simulink model "envModel_rl"  (R2020b)
settings: Solver=ode23t  StartTime=0.0  StopTime=Tf  RelTol=1e-2
values from neighbouring files (symbols this model uses):
  simlen = 100    [main_rl.m]    (also in main_rl_func_modified.m; new_main_rl.m = 80)
  Tf = 200    [RLenv.m]    (also in RlEnvModel.m; demo_rl.m; main_rl.m = simlen*Ts; main_rl_func_modified.m = simlen*Ts)
  Ts = 0.1    [RLenv.m]    (also in RlEnvModel.m; demo_rl.m; main_rl.m = s.Ts; main_rl_func_modified.m = s.Ts)
  ulim = s.actuatorRange    [main_rl.m]    (also in main_rl_func_modified.m; new_main_rl.m)
  whichAg_sim = whichAg_sim*5    (= 30)    [main_rl.m]    (also in main_rl_func_modified.m; new_main_rl.m)
  ylim = s.sensorRange    [main_rl.m]    (also in main_rl_func_modified.m; new_main_rl.m)
undefined symbols (not defined in the file or in its folder): s
libraries: rllib x3, simulink x2
settings Model: Creator=The MathWorks, Inc.  LastModifiedBy=Asus

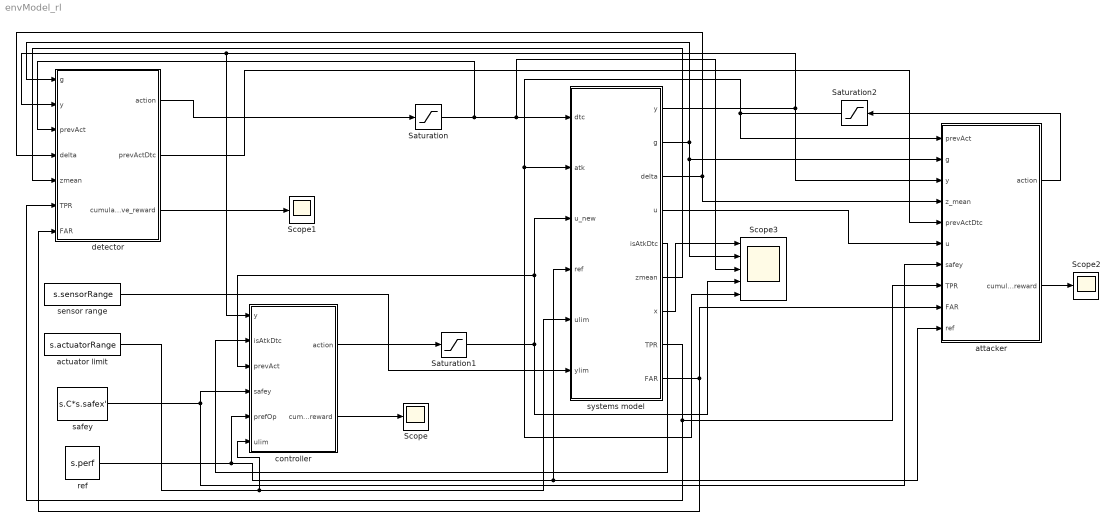
== system envModel_rl ==
  Saturation : Saturate  UpperLimit=[100;simlen]  LowerLimit=[0;1]
  Saturation1 : Saturate  UpperLimit=s.actuatorRange  LowerLimit=-s.actuatorRange
  Saturation2 : Saturate  UpperLimit=[ulim;ylim]  LowerLimit=-[ulim;ylim]
  Scope : Scope
  Scope1 : Scope
  Scope2 : Scope
  Scope3 : Scope  NumInputPorts=5
  actuator limit : Constant  Value=s.actuatorRange
  attacker : Subsystem
  controller : Subsystem
  detector : Subsystem
  ref : Constant  Value=s.perf
  safey : Constant  Value=s.C*s.safex'
  sensor range : Constant  Value=s.sensorRange
  systems model : Subsystem
  wires:
  systems model/1(y) -> controller/1(y), detector/2(y), attacker/3(y)
  ref/1 -> attacker/10(ref), systems model/4(ref), controller/5(prefOp)
  safey/1 -> attacker/7(safey), controller/4(safey)
  systems model/3(delta) -> detector/4(delta), attacker/4(z_mean)
  systems model/2(g) -> detector/1(g), Scope3/2, attacker/2(g)
  sensor range/1 -> systems model/6(ylim)
  actuator limit/1 -> controller/6(ulim), systems model/5(ulim)
  Saturation/1 -> detector/3(prevAct), Scope3/3, systems model/1(dtc)
  Saturation1/1 -> systems model/3(u_new), controller/3(prevAct), Scope3/4
  Saturation2/1 -> attacker/1(prevAct), systems model/2(atk), Scope3/5
  systems model/7(x) -> Scope3/1
  systems model/9(FAR) -> attacker/9(FAR), detector/7(FAR)
  systems model/8(TPR) -> attacker/8(TPR), detector/6(TPR)
  systems model/6(zmean) -> detector/5(zmean)
  detector/1(action) -> Saturation/1
  detector/3(cumulative_reward) -> Scope1/1
  systems model/5(isAtkDtc) -> controller/2(isAtkDtc)
  controller/1(action) -> Saturation1/1
  controller/2(cumulative_reward) -> Scope/1
  detector/2(prevActDtc) -> attacker/5(prevActDtc)
  systems model/4(u) -> attacker/6(u)
  attacker/1(action) -> Saturation2/1
  attacker/2(cumulative_reward) -> Scope2/1

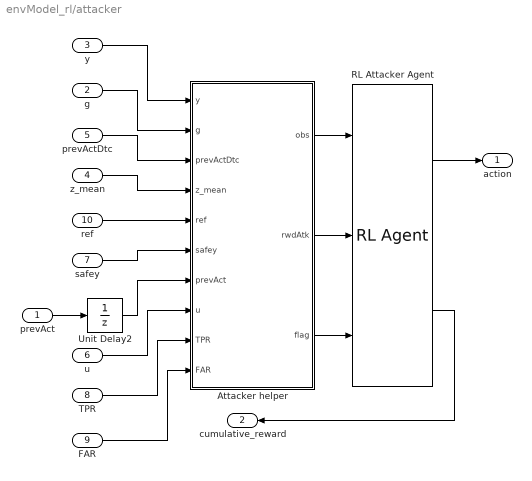
== system envModel_rl/attacker ==
  prevAct : Inport
  g : Inport  Port=2
  y : Inport  Port=3
  z_mean : Inport  Port=4
  prevActDtc : Inport  Port=5
  u : Inport  Port=6
  safey : Inport  Port=7
  TPR : Inport  Port=8
  FAR : Inport  Port=9
  ref : Inport  Port=10
  Attacker helper : Subsystem
  RL Attacker Agent : rllib/RL Agent  Agent=agentAtk  ProvideReward=on  ProvideIsDone=on  ProvideCumRwd=on  TreatAsDirectFeedthrough=on  CollectLoggedSignals=on  CollectModelStates=on
  Unit Delay2 : UnitDelay  SampleTime=-1  HasFrameUpgradeWarning=on
  action : Outport
  cumulative_reward : Outport  Port=2
  wires:
  z_mean/1 -> Attacker helper/4(z_mean)
  prevAct/1 -> Unit Delay2/1
  y/1 -> Attacker helper/1(y)
  ref/1 -> Attacker helper/5(ref)
  Attacker helper/3(flag) -> RL Attacker Agent/3
  Attacker helper/1(obs) -> RL Attacker Agent/1
  Attacker helper/2(rwdAtk) -> RL Attacker Agent/2
  RL Attacker Agent/2 -> cumulative_reward/1
  Unit Delay2/1 -> Attacker helper/7(prevAct)
  RL Attacker Agent/1 -> action/1
  TPR/1 -> Attacker helper/9(TPR)
  FAR/1 -> Attacker helper/10(FAR)
  prevActDtc/1 -> Attacker helper/3(prevActDtc)
  g/1 -> Attacker helper/2(g)
  u/1 -> Attacker helper/8(u)
  safey/1 -> Attacker helper/6(safey)

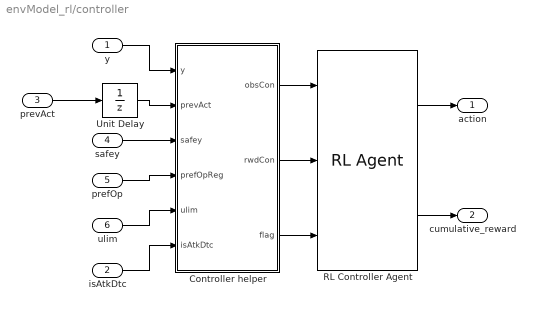
== system envModel_rl/controller ==
  y : Inport
  isAtkDtc : Inport  Port=2
  prevAct : Inport  Port=3
  safey : Inport  Port=4
  prefOp : Inport  Port=5
  ulim : Inport  Port=6
  Controller helper : Subsystem
  RL Controller Agent : rllib/RL Agent  Agent=agentCon  ProvideReward=on  ProvideIsDone=on  ProvideCumRwd=on  TreatAsDirectFeedthrough=on  CollectLoggedSignals=on  CollectModelStates=on
  Unit Delay : UnitDelay  SampleTime=-1  HasFrameUpgradeWarning=on
  action : Outport
  cumulative_reward : Outport  Port=2
  wires:
  Unit Delay/1 -> Controller helper/2(prevAct)
  RL Controller Agent/2 -> cumulative_reward/1
  prefOp/1 -> Controller helper/4(prefOpReg)
  Controller helper/1(obsCon) -> RL Controller Agent/1
  ulim/1 -> Controller helper/5(ulim)
  Controller helper/3(flag) -> RL Controller Agent/3
  safey/1 -> Controller helper/3(safey)
  prevAct/1 -> Unit Delay/1
  Controller helper/2(rwdCon) -> RL Controller Agent/2
  isAtkDtc/1 -> Controller helper/6(isAtkDtc)
  RL Controller Agent/1 -> action/1
  y/1 -> Controller helper/1(y)

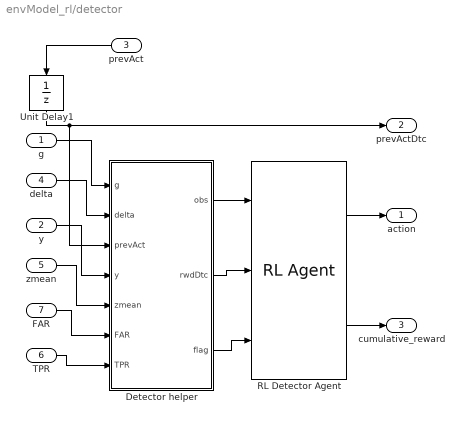
== system envModel_rl/detector ==
  g : Inport
  y : Inport  Port=2
  prevAct : Inport  Port=3
  delta : Inport  Port=4
  zmean : Inport  Port=5
  TPR : Inport  Port=6
  FAR : Inport  Port=7
  Detector helper : Subsystem
  RL Detector Agent : rllib/RL Agent  Agent=agentDtc  ProvideReward=on  ProvideIsDone=on  ProvideCumRwd=on  TreatAsDirectFeedthrough=on  CollectLoggedSignals=on  CollectModelStates=on
  Unit Delay1 : UnitDelay  SampleTime=-1  HasFrameUpgradeWarning=on
  action : Outport
  prevActDtc : Outport  Port=2
  cumulative_reward : Outport  Port=3
  wires:
  FAR/1 -> Detector helper/6(FAR)
  TPR/1 -> Detector helper/7(TPR)
  g/1 -> Detector helper/1(g)
  y/1 -> Detector helper/4(y)
  prevAct/1 -> Unit Delay1/1
  RL Detector Agent/2 -> cumulative_reward/1
  Detector helper/3(flag) -> RL Detector Agent/3
  Detector helper/1(obs) -> RL Detector Agent/1
  Detector helper/2(rwdDtc) -> RL Detector Agent/2
  RL Detector Agent/1 -> action/1
  zmean/1 -> Detector helper/5(zmean)
  delta/1 -> Detector helper/2(delta)
  Unit Delay1/1 -> prevActDtc/1, Detector helper/3(prevAct)

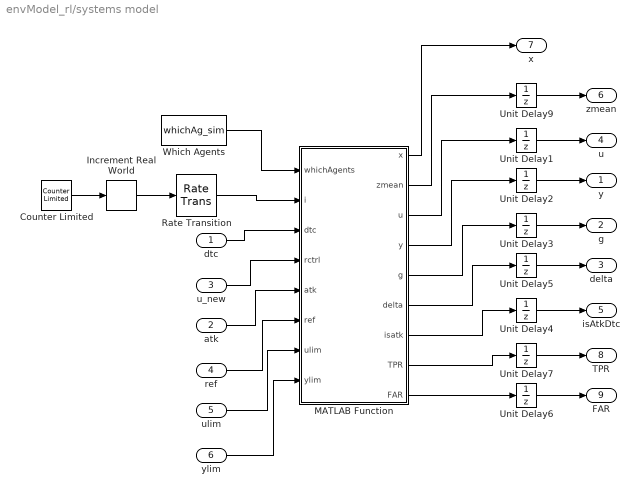
== system envModel_rl/systems model ==
  dtc : Inport
  atk : Inport  Port=2
  u_new : Inport  Port=3
  ref : Inport  Port=4
  ulim : Inport  Port=5
  ylim : Inport  Port=6
  Counter Limited : simulink/Sources/Counter Limited  uplimit=Tf/Ts-2  tsamp=Ts
  Increment Real World : simulink/Additional Math & Discrete/Additional Math: Increment - Decrement/Increment Real World
      settings: SourceProductBaseCode=SL
  MATLAB Function : MATLAB Function  TreatAsAtomicUnit=on
  Rate Transition : RateTransition
  Unit Delay{1..7,9} (8 alike) : UnitDelay  SampleTime=-1  HasFrameUpgradeWarning=on
  Which Agents : Constant  Value=whichAg_sim  SampleTime=Ts
  y : Outport
  g : Outport  Port=2
  delta : Outport  Port=3
  u : Outport  Port=4
  isAtkDtc : Outport  Port=5
  zmean : Outport  Port=6
  x : Outport  Port=7
  TPR : Outport  Port=8
  FAR : Outport  Port=9
  wires:
  Unit Delay9/1 -> zmean/1
  Unit Delay7/1 -> TPR/1
  Unit Delay6/1 -> FAR/1
  Unit Delay2/1 -> y/1
  MATLAB Function/8(TPR) -> Unit Delay7/1
  Unit Delay3/1 -> g/1
  Unit Delay4/1 -> isAtkDtc/1
  Unit Delay5/1 -> delta/1
  Increment Real World/1 -> Rate Transition/1
  Rate Transition/1 -> MATLAB Function/2(i)
  MATLAB Function/5(g) -> Unit Delay3/1
  MATLAB Function/6(delta) -> Unit Delay5/1
  ulim/1 -> MATLAB Function/7(ulim)
  Which Agents/1 -> MATLAB Function/1(whichAgents)
  MATLAB Function/4(y) -> Unit Delay2/1
  Unit Delay1/1 -> u/1
  ref/1 -> MATLAB Function/6(ref)
  ylim/1 -> MATLAB Function/8(ylim)
  Counter Limited/1 -> Increment Real World/1
  MATLAB Function/3(u) -> Unit Delay1/1
  atk/1 -> MATLAB Function/5(atk)
  dtc/1 -> MATLAB Function/3(dtc)
  MATLAB Function/7(isatk) -> Unit Delay4/1
  u_new/1 -> MATLAB Function/4(rctrl)
  MATLAB Function/1(x) -> x/1
  MATLAB Function/2(zmean) -> Unit Delay9/1
  MATLAB Function/9(FAR) -> Unit Delay6/1

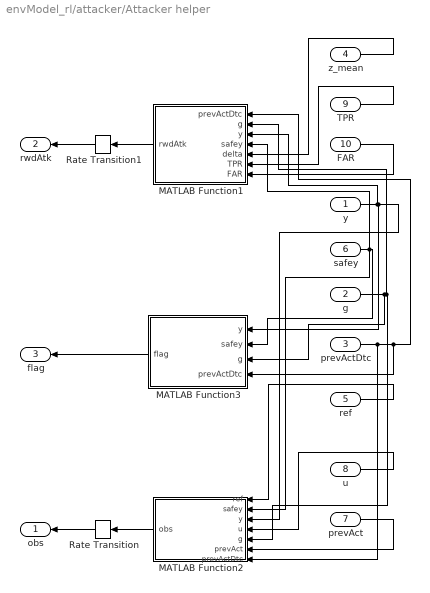
== system envModel_rl/attacker/Attacker helper ==
  y : Inport
  g : Inport  Port=2
  prevActDtc : Inport  Port=3
  z_mean : Inport  Port=4
  ref : Inport  Port=5
  safey : Inport  Port=6
  prevAct : Inport  Port=7
  u : Inport  Port=8
  TPR : Inport  Port=9
  FAR : Inport  Port=10
  MATLAB Function1 : MATLAB Function  TreatAsAtomicUnit=on
  MATLAB Function2 : MATLAB Function  TreatAsAtomicUnit=on
  MATLAB Function3 : MATLAB Function  TreatAsAtomicUnit=on
  Rate Transition : RateTransition
  Rate Transition1 : RateTransition
  obs : Outport
  rwdAtk : Outport  Port=2
  flag : Outport  Port=3
  wires:
  MATLAB Function1/1(rwdAtk) -> Rate Transition1/1
  ref/1 -> MATLAB Function2/1(ref)
  z_mean/1 -> MATLAB Function1/5(delta)
  prevAct/1 -> MATLAB Function2/6(prevAct)
  u/1 -> MATLAB Function2/4(u)
  TPR/1 -> MATLAB Function1/6(TPR)
  MATLAB Function3/1(flag) -> flag/1
  FAR/1 -> MATLAB Function1/7(FAR)
  Rate Transition/1 -> obs/1
  safey/1 -> MATLAB Function1/4(safey), MATLAB Function2/2(safey), MATLAB Function3/2(safey)
  MATLAB Function2/1(obs) -> Rate Transition/1
  Rate Transition1/1 -> rwdAtk/1
  prevActDtc/1 -> MATLAB Function3/4(prevActDtc), MATLAB Function1/1(prevActDtc), MATLAB Function2/7(prevActDtc)
  y/1 -> MATLAB Function2/3(y), MATLAB Function3/1(y), MATLAB Function1/3(y)
  g/1 -> MATLAB Function2/5(g), MATLAB Function1/2(g), MATLAB Function3/3(g)

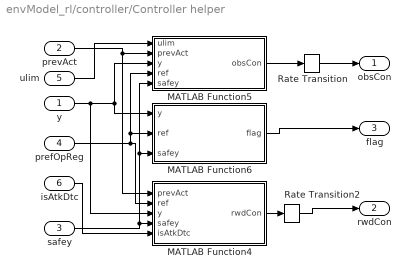
== system envModel_rl/controller/Controller helper ==
  y : Inport
  prevAct : Inport  Port=2
  safey : Inport  Port=3
  prefOpReg : Inport  Port=4
  ulim : Inport  Port=5
  isAtkDtc : Inport  Port=6
  MATLAB Function4 : MATLAB Function  TreatAsAtomicUnit=on
  MATLAB Function5 : MATLAB Function  TreatAsAtomicUnit=on
  MATLAB Function6 : MATLAB Function  TreatAsAtomicUnit=on
  Rate Transition : RateTransition
  Rate Transition2 : RateTransition
  obsCon : Outport
  rwdCon : Outport  Port=2
  flag : Outport  Port=3
  wires:
  prefOpReg/1 -> MATLAB Function6/2(ref), MATLAB Function5/4(ref), MATLAB Function4/2(ref)
  safey/1 -> MATLAB Function5/5(safey), MATLAB Function6/3(safey), MATLAB Function4/4(safey)
  MATLAB Function4/1(rwdCon) -> Rate Transition2/1
  MATLAB Function5/1(obsCon) -> Rate Transition/1
  y/1 -> MATLAB Function6/1(y), MATLAB Function5/3(y), MATLAB Function4/3(y)
  prevAct/1 -> MATLAB Function4/1(prevAct), MATLAB Function5/2(prevAct)
  Rate Transition/1 -> obsCon/1
  MATLAB Function6/1(flag) -> flag/1
  ulim/1 -> MATLAB Function5/1(ulim)
  Rate Transition2/1 -> rwdCon/1
  isAtkDtc/1 -> MATLAB Function4/5(isAtkDtc)

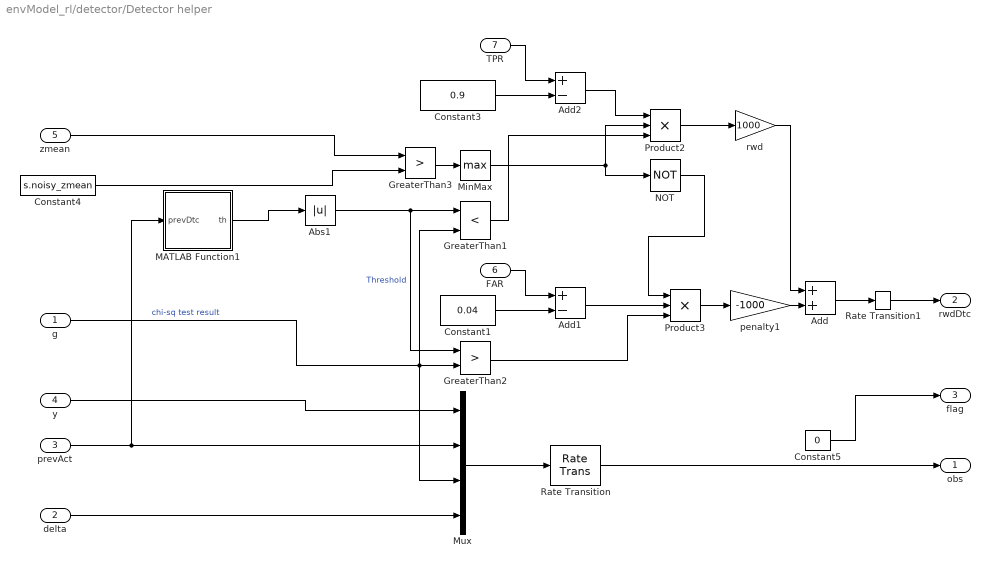
== system envModel_rl/detector/Detector helper ==
  g : Inport
  delta : Inport  Port=2
  prevAct : Inport  Port=3
  y : Inport  Port=4
  zmean : Inport  Port=5
  FAR : Inport  Port=6
  TPR : Inport  Port=7
  Abs1 : Abs
  Add : Sum
  Add1 : Sum  Inputs=+-
  Add2 : Sum  Inputs=+-
  Constant1 : Constant  Value=0.04  SampleTime=Ts
  Constant3 : Constant  Value=0.9  SampleTime=Ts
  Constant4 : Constant  Value=s.noisy_zmean  SampleTime=Ts
  Constant5 : Constant  Value=0  SampleTime=Ts
  GreaterThan1 : RelationalOperator  Operator=<  OutDataTypeStr=boolean  RndMeth=Simplest
  GreaterThan2 : RelationalOperator  Operator=>  OutDataTypeStr=boolean  RndMeth=Simplest
  GreaterThan3 : RelationalOperator  Operator=>  OutDataTypeStr=boolean  RndMeth=Simplest
  MATLAB Function1 : MATLAB Function  TreatAsAtomicUnit=on
  MinMax : MinMax  Function=max
  Mux : Mux
  NOT : Logic  Operator=NOT  IconShape=distinctive  AllPortsSameDT=off  OutDataTypeStr=boolean
  Product2 : Product  Inputs=3
  Product3 : Product  Inputs=3
  Rate Transition : RateTransition
  Rate Transition1 : RateTransition
  penalty1 : Gain  Gain=-1000
  rwd : Gain  Gain=1000
  obs : Outport
  rwdDtc : Outport  Port=2
  flag : Outport  Port=3
  wires:
  GreaterThan1/1 -> Product2/3
  GreaterThan2/1 -> Product3/3
  NOT/1 -> Product3/1
  Constant5/1 -> flag/1
  y/1 -> Mux/1
  Product3/1 -> penalty1/1
  Abs1/1 -> GreaterThan1/1, GreaterThan2/1  "Threshold"
  Add1/1 -> Product3/2
  Add2/1 -> Product2/1
  Product2/1 -> rwd/1
  Rate Transition/1 -> obs/1
  Constant3/1 -> Add2/2
  prevAct/1 -> MATLAB Function1/1(prevDtc), Mux/2
  delta/1 -> Mux/4
  Mux/1 -> Rate Transition/1
  Rate Transition1/1 -> rwdDtc/1
  Constant1/1 -> Add1/2
  TPR/1 -> Add2/1
  FAR/1 -> Add1/1
  MATLAB Function1/1(th) -> Abs1/1
  rwd/1 -> Add/1
  Add/1 -> Rate Transition1/1
  GreaterThan3/1 -> MinMax/1
  g/1 -> GreaterThan2/2, Mux/3, GreaterThan1/2  "chi-sq test result"
  penalty1/1 -> Add/2
  zmean/1 -> GreaterThan3/1
  Constant4/1 -> GreaterThan3/2
  MinMax/1 -> NOT/1, Product2/2

== matlab function envModel_rl/controller/Controller helper/MATLAB Function6 ==
  data: y input; ref input; flag output; safey input
function flag = stop(y,ref,safey)
flag= 0;
% flag = abs((y-ref)/ref) <= 0.25;

== matlab function envModel_rl/detector/Detector helper/MATLAB Function1 ==
  data: prevDtc input; th output
function th   = split(prevDtc)
%    format long g;
   th = prevDtc(1);
    l = prevDtc(2);
end

== matlab function envModel_rl/attacker/Attacker helper/MATLAB Function1 ==
  data: rwdAtk output; prevActDtc input; g input; y input; safey input; delta input; TPR input; FAR input
function rwdAtk  = rwrdAtk(prevActDtc,g,y,safey,delta,TPR,FAR)
%    format long g;
   th = abs(prevActDtc(1));
   tau = max(1,ceil(prevActDtc(2,1)));
   dof = size(y,1)*(tau);
%    FAR = chi2cdf(th,dof,'upper')
%    TPR = ncx2cdf(th,dof,abs(delta),'upper');
%    rwdAtk = FAR/TPR + 50*(g<th)+ 100*(y-ref)^2;
%             50*(FAR-0.05)-40*TPR + 50*(g<th)+ 100*(abs(y)-abs(safey))
% % rwdAtk = 50*(1-FAR) -50*TPR + 100*(g<th & abs(y)>abs(safey))+ 100*(abs(y)-abs(safey))
% rwdAtk = 50*(-FAR) -50*TPR + 100*(g<th)*(abs(y)-abs(safey))+ 100*(g<th)*(abs(y)-0.4*abs(safey))
rwdAtk = 500*(FAR) -1000*TPR + 1000*(g<th)*max(abs(y)-0.3*abs(safey))+1000*(th-g)

== matlab function envModel_rl/systems model/MATLAB Function ==
  data: x output; zmean output; whichAgents input; u output; i input; y output; g output; delta output; dtc input; rctrl input; atk input; ref input; ulim input; ylim input; s parameter; isatk output; TPR output; FAR output
function [x,zmean,u,y,g,delta,isatk,TPR,FAR] = env(whichAgents,i,dtc,rctrl,atk,ref,ulim,ylim, s)
% function [y,g,z_mean]= envSys(atk,dtc,new_u,ref, s)
xdim= size(s.A,2);
ydim= size(s.C,1);
udim= size(s.B,2);
au=zeros(udim,1);
ay=zeros(ydim,1);
%% SYS_ENV progress every iteration goes here
if ~rem(whichAgents,2)
    disp("with attacker agent");
    for i1=1:udim
        au(i1,1)= atk(i1,1);
    end
    for i2=1:udim
        ay(i2,1)= atk(udim+i2,1);
    end  
else
    disp("without attacker agent, no attack, only noise");
    au=zeros(udim,1);
    ay=zeros(ydim,1);
end
% 3 for controller agent
if ~rem(whichAgents,3)
    u_new= rctrl;
    disp("with controller agent");
else
    u_new = zeros(size(rctrl));
    disp("without controller agent, with default control action");
end
% 5 for detector agent
if ~rem(whichAgents,5)
    th= abs(dtc(1));
    dtc_windw= max(1,(ceil(dtc(2))));
    disp("with detector agent");
else
    disp("without detector agent, with default threshold, dof");
    th=s.th;
    dtc_windw=1;
end

            s.t(i+1)=s.t(i)+s.Ts;
            s.a_u(:,i+1)=au.*s.uatkon;
            s.a_y(:,i+1)=ay.*s.yatkon;
            s.x_act(:,i+1) = s.A*s.x_act(:,i)+s.B*s.uatk(:,i)+s.proc_noise(:,i);
%             s.xatk(i)= s.A*s.x_act(i)+s.B*s.u_act(i);
            s.xhat(:,i+1) = s.A*s.xhat(:,i) + s.B*s.u_act(:,i) + s.L*s.z(:,i);
            s.est_err(:,i+1)= s.x_act(:,i+1)-s.xhat(:,i+1);
            s.u_act(:,i+1)= max(-ulim,min(ulim,s.K*s.xhat(:,i+1)));
            s.uatk(:,i+1)= max(-ulim,min(ulim,s.u_act(:,i+1)+s.a_u(:,i+1)));
            s.y_act(:,i+1)= max(-ylim,min(ylim,s.C*s.x_act(:,i+1))+s.meas_noise(:,i));
            s.yatk(:,i+1)= max(-ylim,min(ylim,s.y_act(:,i+1)+s.a_y(:,i+1)));
            s.z(:,i+1)= s.yatk(:,i+1)-s.C*s.xhat(:,i+1);
            for i3=1:size(s.z,1)
                z_current=s.z(i3,1:i)';
                s.z_mean(i3,i+1)= mean(z_current)';
                s.z_var(i3,i+1) = var(z_current)';
                
            end
            z_covar = cov( s.z(:,1:i+1)');
%             if det(z_covar)==0
%                 s.z_var(:,i+1)=s.z_var(:,i);
%                 disp("singular")
%             end
            s.chi_tst(i+1)= s.z(:,i+1)'*inv(s.noisy_zvar)*s.z(:,i+1); % ttc without noise z var=0.1
%             s.chi_tst(i+1)= s.z(:,i+1)'*inv(cov(s.z'))*s.z(:,i+1);
             if ~isfinite(s.chi_tst(i+1))
                    s.chi_tst(i+1)= 0;
             end
            s.threshold(i+1)= th;
            s.tau(i+1)= dtc_windw;
            s.g(i+1) = 0;       
            s.non_cent(:,i+1)= 0;
%             if i-tau+1 > 0                  % Calculate detector window starting index
%                 srt = i-tau+1;              % tau is the detector window length
%             else
%                 srt = 1;
%             end
%% Chi square test and non centrality calculation
            for k = max(1,i-s.tau(i+1)+1):i
                
                s.g(i+1) = s.g(i+1) + s.chi_tst(k+1);  % Calculate gk (chi2 test)
                del= s.z_mean(:,k+1)'*inv(z_covar)*s.z_mean(:,k+1);
%                 del= s.z_mean(:,k+1)'*inv(cov(s.z'))*s.z_mean(:,k+1);
                if ~isfinite(inv(z_covar))
                    s.non_cent(i+1)= s.non_cent(i+1) + 0;
                else
                    s.non_cent(i+1)= s.non_cent(i+1) + del;
                end
            end
            
%% to start the RL based controller
            if (max(abs(s.yatk(i+1))>abs(ref*s.C*s.safex'))) || (s.g(i+1) > s.threshold(i+1))
                s.u_act(:,i+1) = max(-ulim,min(ulim,u_new));
                s.uatk(:,i+1)= max(-ulim,min(ulim,s.u_act(:,i+1)+s.a_u(:,i+1)));
                isatk=1;
                disp("detected");
%                 plot(s.yatk);
%                 hold on;
%                 plot(s.z');
%                 hold on;
%                 plot(s.g');
%                 hold on;
%                 plot(s.threshold');
%                 hold on;
%                 plot((s.safex*ones(size(s.A,1),size(s.t,2)))');
%                 hold on;
%                 plot((s.safex*ones(size(s.A,1),size(s.t,2)))');
%                 hold off;
            else
                isatk=0;
            end
            
    disp("iteration: "+i)
    th= s.threshold(i+1)
    window= s.tau(i+1)
    dof= s.tau(i+1)*size(s.C,1)
    TPR= ncx2cdf(s.threshold(i+1),dof,s.non_cent(i+1),'upper')
    FAR= chi2cdf(s.threshold(i+1),dof,'upper')
    s.avgtpr(i+1)= TPR;
    s.avgfar(i+1)= FAR;
    avgtpr= mean(s.avgtpr)
    avgfar= mean(s.avgfar)
    g= s.g(i+1)
    y=s.yatk(:,i+1)
    u=s.uatk(:,i+1)
    delta = s.non_cent(i+1)
    fdi=[ay;au]
    x=s.x_act(:,i+1)
    zmean=s.z_mean(:,i+1)
end

== matlab function envModel_rl/attacker/Attacker helper/MATLAB Function2 ==
  data: obs output; ref input; safey input; y input; u input; g input; prevAct input; prevActDtc input
function obs = obsAtk(ref,safey,y,u,g,prevAct,prevActDtc)
%     format long g;
    ay= prevAct(1,1);
    au= prevAct(2,1);
    obs= [ref;y-ay;u-au;g;safey;prevAct;prevActDtc];

== matlab function envModel_rl/attacker/Attacker helper/MATLAB Function3 ==
  data: y input; flag output; safey input; g input; prevActDtc input
function flag  = stop(y,safey, g, prevActDtc)
%     format long g;
    th = abs(prevActDtc(1));
%     flag = y > safey & g <= th;
flag=0;

== matlab function envModel_rl/controller/Controller helper/MATLAB Function4 ==
  data: rwdCon output; prevAct input; ref input; y input; safey input; isAtkDtc input
function rwdCon  = rwrdCon(prevAct,ref,y,safey,isAtkDtc)
%     format long g;
    u=prevAct;
%     ay=atk(2);
    %% safer : 0.5* safey
%     rwdCon = 350*(abs((y-ref)/ref) <= 0.30)-20*(prevAct)^2-100*(abs(y) > safey)-50
rwdCon = isAtkDtc*(-(y-ref*safey)'*1000*(y-ref*safey))%-20*u^2

== matlab function envModel_rl/controller/Controller helper/MATLAB Function5 ==
  data: ulim input; obsCon output; prevAct input; y input; ref input; safey input
function obsCon = obsCon(ulim,prevAct,y,ref,safey)
   
    obsCon=[ulim;prevAct;y;ref;safey];
